simulink model "AttitudePID"  (R2019b)
settings: Solver=VariableStepAuto  StartTime=0.0  StopTime=500  RelTol=1e-3
libraries: simulink x3
settings Model: Creator=80741  LastModifiedBy=80741

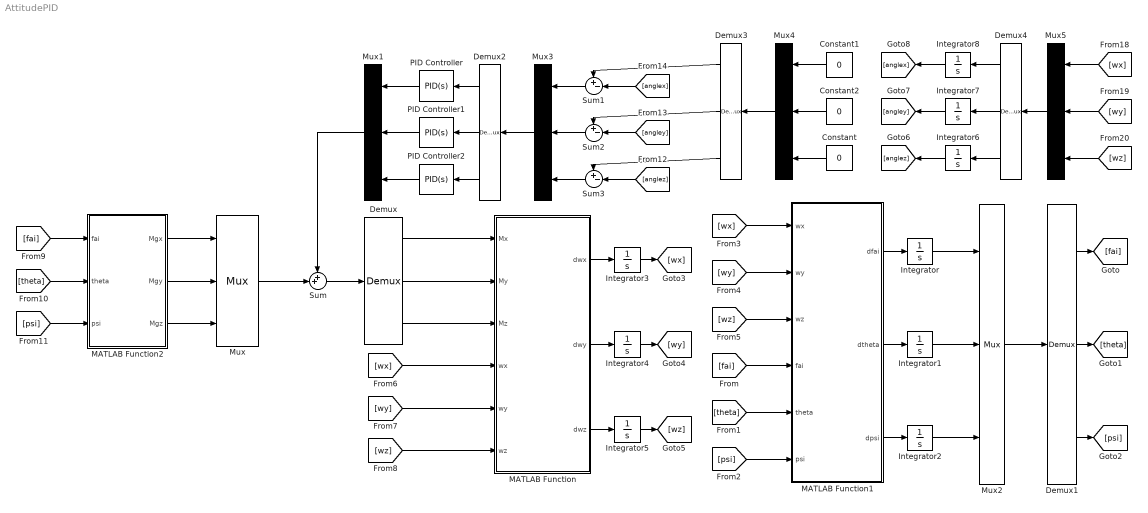
== system AttitudePID ==
  Constant : Constant  Value=0
  Constant1 : Constant  Value=0
  Constant2 : Constant  Value=0
  Demux{,1..4} (5 alike) : Demux  Outputs=3
  Integrator : Integrator  InitialCondition=5
  Integrator{1..2,5..8} (6 alike) : Integrator
  Integrator3 : Integrator  InitialCondition=0.04
  Integrator4 : Integrator  InitialCondition=0.08
  MATLAB Function : MATLAB Function  TreatAsAtomicUnit=on
  MATLAB Function1 : MATLAB Function  TreatAsAtomicUnit=on
  MATLAB Function2 : MATLAB Function  TreatAsAtomicUnit=on
  Mux{,1..5} (6 alike) : Mux  Inputs=3
  PID Controller : simulink/Continuous/PID Controller  Controller=PID  Form=Parallel  TimeDomain=Continuous-time  SampleTime=-1  IntegratorMethod=Forward Euler  FilterMethod=Forward Euler  ControllerParametersSource=internal  P=0.852201667952021  I=0.182203588363595  D=47.6922615532766  UseFilter=on  N=0.109217462973731  TunerSelectOption=Transfer Function Based (PID Tuner App)  InitialConditionSource=internal  InitialConditionForIntegrator=0  InitialConditionForFilter=0  DifferentiatorICPrevScaledInput=0  ExternalReset=none  TrackingMode=off  Kt=1  LimitOutput=off  UpperSaturationLimit=inf  LowerSaturationLimit=-inf  LinearizeAsGain=on  AntiWindupMode=none  Kb=1  POutMin=[]  POutMax=[]  IOutMin=[]  IOutMax=[]  DOutMin=[]  DOutMax=[]  NOutMin=[]  NOutMax=[]  SumOutMin=[]  SumOutMax=[]  SaturationOutMin=[]  SaturationOutMax=[]  PParamMin=[]  PParamMax=[]  IParamMin=[]  IParamMax=[]  DParamMin=[]  DParamMax=[]  NParamMin=[]  NParamMax=[]  KbParamMin=[]  KbParamMax=[]  KtParamMin=[]  KtParamMax=[]  KbOutMin=[]  KbOutMax=[]  KtOutMin=[]  KtOutMax=[]  IntegratorOutMin=[]  IntegratorOutMax=[]  FilterOutMin=[]  FilterOutMax=[]  SumI1OutMin=[]  SumI1OutMax=[]  SumI2OutMin=[]  SumI2OutMax=[]  SumI3OutMin=[]  SumI3OutMax=[]  SumI4OutMin=[]  SumI4OutMax=[]  SumDOutMin=[]  SumDOutMax=[]  DifferentiatorOutMin=[]  DifferentiatorOutMax=[]  FilterDiffOutCoefMin=[]  FilterDiffOutCoefMax=[]  ReciprocalOutMin=[]  ReciprocalOutMax=[]  SumDenOutMin=[]  SumDenOutMax=[]  SumNumOutMin=[]  SumNumOutMax=[]  DivideOutMin=[]  DivideOutMax=[]  IntegratorContinuousStateAttributes=''  IntegratorStateMustResolveToSignalObject=off  IntegratorRTWStateStorageClass=Auto  FilterContinuousStateAttributes=''  FilterStateMustResolveToSignalObject=off  FilterRTWStateStorageClass=Auto  ParallelPVariant=InternalParameters  IdealPVariant=Disabled  IVariant=InternalParameters  DVariant=InternalParameters  IntegratorVariant=Continuous  SatVariant=Disabled  AWVariant=Passthrough  PCopyVariant=Disabled  TRVariant=Disabled  FdbkBlocksVariant=Forward  IdealPFdbkVariant=Disabled  SatFdbkVariant=Disabled  DerivativeFilterVariant=ContFilter  NVariant=InternalParameters  NCopyVariant=Disabled  FilterICVariant=InternalICsFilter  IntegratorICVariant=InternalICs  ExternalResetVariant=Disabled  TRSumVariant=Passthrough  SumFdbkVariant=Disabled  SumVariant=Sum_PID
  PID Controller1 : simulink/Continuous/PID Controller  Controller=PID  Form=Parallel  TimeDomain=Continuous-time  SampleTime=-1  IntegratorMethod=Forward Euler  FilterMethod=Forward Euler  ControllerParametersSource=internal  P=0.728529840117402  I=0.0105769015571864  D=14.0861012139973  UseFilter=on  N=0.12050837606086  TunerSelectOption=Transfer Function Based (PID Tuner App)  InitialConditionSource=internal  InitialConditionForIntegrator=0  InitialConditionForFilter=0  DifferentiatorICPrevScaledInput=0  ExternalReset=none  TrackingMode=off  Kt=1  LimitOutput=off  UpperSaturationLimit=inf  LowerSaturationLimit=-inf  LinearizeAsGain=on  AntiWindupMode=none  Kb=1  POutMin=[]  POutMax=[]  IOutMin=[]  IOutMax=[]  DOutMin=[]  DOutMax=[]  NOutMin=[]  NOutMax=[]  SumOutMin=[]  SumOutMax=[]  SaturationOutMin=[]  SaturationOutMax=[]  PParamMin=[]  PParamMax=[]  IParamMin=[]  IParamMax=[]  DParamMin=[]  DParamMax=[]  NParamMin=[]  NParamMax=[]  KbParamMin=[]  KbParamMax=[]  KtParamMin=[]  KtParamMax=[]  KbOutMin=[]  KbOutMax=[]  KtOutMin=[]  KtOutMax=[]  IntegratorOutMin=[]  IntegratorOutMax=[]  FilterOutMin=[]  FilterOutMax=[]  SumI1OutMin=[]  SumI1OutMax=[]  SumI2OutMin=[]  SumI2OutMax=[]  SumI3OutMin=[]  SumI3OutMax=[]  SumI4OutMin=[]  SumI4OutMax=[]  SumDOutMin=[]  SumDOutMax=[]  DifferentiatorOutMin=[]  DifferentiatorOutMax=[]  FilterDiffOutCoefMin=[]  FilterDiffOutCoefMax=[]  ReciprocalOutMin=[]  ReciprocalOutMax=[]  SumDenOutMin=[]  SumDenOutMax=[]  SumNumOutMin=[]  SumNumOutMax=[]  DivideOutMin=[]  DivideOutMax=[]  IntegratorContinuousStateAttributes=''  IntegratorStateMustResolveToSignalObject=off  IntegratorRTWStateStorageClass=Auto  FilterContinuousStateAttributes=''  FilterStateMustResolveToSignalObject=off  FilterRTWStateStorageClass=Auto  ParallelPVariant=InternalParameters  IdealPVariant=Disabled  IVariant=InternalParameters  DVariant=InternalParameters  IntegratorVariant=Continuous  SatVariant=Disabled  AWVariant=Passthrough  PCopyVariant=Disabled  TRVariant=Disabled  FdbkBlocksVariant=Forward  IdealPFdbkVariant=Disabled  SatFdbkVariant=Disabled  DerivativeFilterVariant=ContFilter  NVariant=InternalParameters  NCopyVariant=Disabled  FilterICVariant=InternalICsFilter  IntegratorICVariant=InternalICs  ExternalResetVariant=Disabled  TRSumVariant=Passthrough  SumFdbkVariant=Disabled  SumVariant=Sum_PID
  PID Controller2 : simulink/Continuous/PID Controller  Controller=PID  Form=Parallel  TimeDomain=Continuous-time  SampleTime=-1  IntegratorMethod=Forward Euler  FilterMethod=Forward Euler  ControllerParametersSource=internal  P=2.7388432502212  I=3.30295754342705e-07  D=26.5610990403586  UseFilter=on  N=75.1925414097897  TunerSelectOption=Transfer Function Based (PID Tuner App)  InitialConditionSource=internal  InitialConditionForIntegrator=0  InitialConditionForFilter=0  DifferentiatorICPrevScaledInput=0  ExternalReset=none  TrackingMode=off  Kt=1  LimitOutput=off  UpperSaturationLimit=inf  LowerSaturationLimit=-inf  LinearizeAsGain=on  AntiWindupMode=none  Kb=1  POutMin=[]  POutMax=[]  IOutMin=[]  IOutMax=[]  DOutMin=[]  DOutMax=[]  NOutMin=[]  NOutMax=[]  SumOutMin=[]  SumOutMax=[]  SaturationOutMin=[]  SaturationOutMax=[]  PParamMin=[]  PParamMax=[]  IParamMin=[]  IParamMax=[]  DParamMin=[]  DParamMax=[]  NParamMin=[]  NParamMax=[]  KbParamMin=[]  KbParamMax=[]  KtParamMin=[]  KtParamMax=[]  KbOutMin=[]  KbOutMax=[]  KtOutMin=[]  KtOutMax=[]  IntegratorOutMin=[]  IntegratorOutMax=[]  FilterOutMin=[]  FilterOutMax=[]  SumI1OutMin=[]  SumI1OutMax=[]  SumI2OutMin=[]  SumI2OutMax=[]  SumI3OutMin=[]  SumI3OutMax=[]  SumI4OutMin=[]  SumI4OutMax=[]  SumDOutMin=[]  SumDOutMax=[]  DifferentiatorOutMin=[]  DifferentiatorOutMax=[]  FilterDiffOutCoefMin=[]  FilterDiffOutCoefMax=[]  ReciprocalOutMin=[]  ReciprocalOutMax=[]  SumDenOutMin=[]  SumDenOutMax=[]  SumNumOutMin=[]  SumNumOutMax=[]  DivideOutMin=[]  DivideOutMax=[]  IntegratorContinuousStateAttributes=''  IntegratorStateMustResolveToSignalObject=off  IntegratorRTWStateStorageClass=Auto  FilterContinuousStateAttributes=''  FilterStateMustResolveToSignalObject=off  FilterRTWStateStorageClass=Auto  ParallelPVariant=InternalParameters  IdealPVariant=Disabled  IVariant=InternalParameters  DVariant=InternalParameters  IntegratorVariant=Continuous  SatVariant=Disabled  AWVariant=Passthrough  PCopyVariant=Disabled  TRVariant=Disabled  FdbkBlocksVariant=Forward  IdealPFdbkVariant=Disabled  SatFdbkVariant=Disabled  DerivativeFilterVariant=ContFilter  NVariant=InternalParameters  NCopyVariant=Disabled  FilterICVariant=InternalICsFilter  IntegratorICVariant=InternalICs  ExternalResetVariant=Disabled  TRSumVariant=Passthrough  SumFdbkVariant=Disabled  SumVariant=Sum_PID
  Sum : Sum  Inputs=++|
  Sum1 : Sum  Inputs=+-|
  Sum2 : Sum  Inputs=+-|
  Sum3 : Sum  Inputs=+-|
  wires:
  MATLAB Function/1(dwx) -> Integrator3/1
  MATLAB Function/2(dwy) -> Integrator4/1
  MATLAB Function/3(dwz) -> Integrator5/1
  MATLAB Function1/1(dfai) -> Integrator/1
  MATLAB Function1/2(dtheta) -> Integrator1/1
  MATLAB Function1/3(dpsi) -> Integrator2/1
  [fai] -> MATLAB Function1/4(fai)
  [theta] -> MATLAB Function1/5(theta)
  [psi] -> MATLAB Function1/6(psi)
  Integrator3/1 -> [wx]
  Integrator4/1 -> [wy]
  Integrator5/1 -> [wz]
  [wx] -> MATLAB Function1/1(wx)
  [wy] -> MATLAB Function1/2(wy)
  [wz] -> MATLAB Function1/3(wz)
  [wx] -> MATLAB Function/4(wx)
  [wy] -> MATLAB Function/5(wy)
  [wz] -> MATLAB Function/6(wz)
  [fai] -> MATLAB Function2/1(fai)
  [theta] -> MATLAB Function2/2(theta)
  [psi] -> MATLAB Function2/3(psi)
  MATLAB Function2/1(Mgx) -> Mux/1
  MATLAB Function2/2(Mgy) -> Mux/2
  MATLAB Function2/3(Mgz) -> Mux/3
  Mux1/1 -> Sum/1
  Sum/1 -> Demux/1
  Demux/1 -> MATLAB Function/1(Mx)
  Demux/2 -> MATLAB Function/2(My)
  Demux/3 -> MATLAB Function/3(Mz)
  Mux/1 -> Sum/2
  PID Controller/1 -> Mux1/1
  PID Controller1/1 -> Mux1/2
  PID Controller2/1 -> Mux1/3
  Integrator/1 -> Mux2/1
  Integrator1/1 -> Mux2/2
  Integrator2/1 -> Mux2/3
  Mux2/1 -> Demux1/1
  Demux1/1 -> [fai]
  Demux1/2 -> [theta]
  Demux1/3 -> [psi]
  Demux2/2 -> PID Controller1/1
  Mux3/1 -> Demux2/1
  Demux2/1 -> PID Controller/1
  Demux2/3 -> PID Controller2/1
  Sum1/1 -> Mux3/1
  Sum2/1 -> Mux3/2
  Sum3/1 -> Mux3/3
  Constant/1 -> Mux4/3
  Constant2/1 -> Mux4/2
  Constant1/1 -> Mux4/1
  Mux4/1 -> Demux3/1
  Demux3/1 -> Sum1/1
  Demux3/2 -> Sum2/1
  Demux3/3 -> Sum3/1
  [wx] -> Mux5/1
  [wy] -> Mux5/2
  [wz] -> Mux5/3
  Mux5/1 -> Demux4/1
  Demux4/1 -> Integrator8/1
  Demux4/2 -> Integrator7/1
  Demux4/3 -> Integrator6/1
  Integrator6/1 -> [anglez]
  Integrator7/1 -> [angley]
  Integrator8/1 -> [anglex]
  [anglez] -> Sum3/2
  [angley] -> Sum2/2
  [anglex] -> Sum1/2

== matlab function AttitudePID/MATLAB Function1 ==
  data: wx input; dfai output; wy input; wz input; fai input; theta input; psi input; dtheta output; dpsi output
function [dfai,dtheta,dpsi] = fcn(wx,wy,wz,fai,theta,psi)
wo=7.292*10^-5;
dfai=wx*cos(theta)+...
    wz*sin(theta)+wo*sin(psi);
dtheta=wy-tan(fai)*(wz*cos(theta)-...
    wx*sin(theta))+wo*cos(psi)/cos(fai);
dpsi=((wz*cos(theta)-wx*sin(theta))...
    -wo*sin(fai)*cos(psi))/cos(fai);

== matlab function AttitudePID/MATLAB Function ==
  data: Mx input; dwx output; My input; Mz input; wx input; wy input; wz input; dwy output; dwz output
function [dwx,dwy,dwz] = fcn(Mx,My,Mz,wx,wy,wz)
Ix=293.375;
Iy=293.375;
Iz=330.75;

dwx=(Mx-wy*wz*(Iz-Iy))/Ix;
dwy=(My-wz*wx*(Ix-Iz))/Iy;
dwz=(Mz-wx*wy*(Iy-Ix))/Iz;

== matlab function AttitudePID/MATLAB Function2 ==
  data: fai input; Mgx output; theta input; psi input; Mgy output; Mgz output
function [Mgx,Mgy,Mgz] = fcn(fai,theta,psi)
Ix=293.375;
Iy=293.375;
Iz=330.75;
wo=7.292*10^-5;

Mgx=1.5*wo^2*(Iz-Iy)*cos(theta)*sin(2*fai);
Mgy=1.5*wo^2*(Iz-Ix)*sin(theta*2)*cos(fai)^2;
Mgz=1.5*wo^2*(Ix-Iy)*sin(theta)*sin(2*fai);
